simulink model "Q3"  (R2018b)
settings: Solver=FixedStepDiscrete  StartTime=0.0  StopTime=0.1  FixedStep=1e-6  RelTol=1e-3
libraries: powerlib x16
settings Model: Creator=canbe  LastModifiedBy=canbe

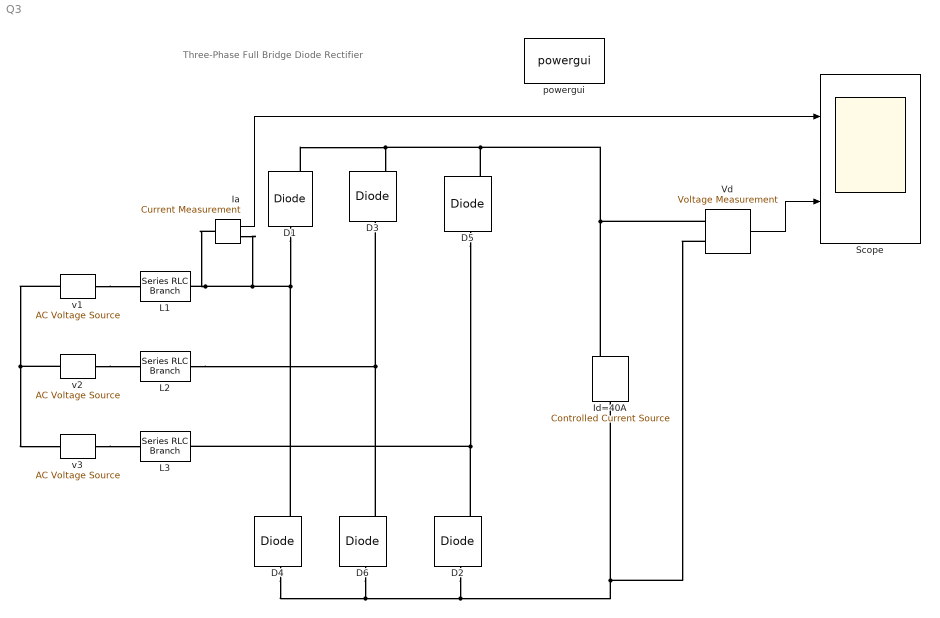
== system Q3 ==
  note: Three-Phase Full Bridge Diode Rectifier
  "D1 " : powerlib/Power Electronics/Diode  Ron=0.001  Lon=0  Vf=0.8  IC=0  UseSnubber=0  Rs=500  Cs=250e-9  Measurements=on
  D2 : powerlib/Power Electronics/Diode  Ron=1e-2  Lon=0  Vf=0.8  IC=0  UseSnubber=off  Rs=1000  Cs=0.1e-6  Measurements=on
      settings: SourceProductName=Simscape Electrical
  "D3 " : powerlib/Power Electronics/Diode  Ron=1e-2  Lon=0  Vf=0.8  IC=0  UseSnubber=off  Rs=1000  Cs=0.1e-6  Measurements=on
      settings: SourceProductName=Simscape Electrical
  "D4 " : powerlib/Power Electronics/Diode  Ron=1e-2  Lon=0  Vf=0.8  IC=0  UseSnubber=off  Rs=1000  Cs=0.1e-6  Measurements=on
      settings: SourceProductName=Simscape Electrical
  "D5 " : powerlib/Power Electronics/Diode  Ron=1e-2  Lon=0  Vf=0.8  IC=0  UseSnubber=off  Rs=1000  Cs=0.1e-6  Measurements=on
      settings: SourceProductName=Simscape Electrical
  D6 : powerlib/Power Electronics/Diode  Ron=1e-2  Lon=0  Vf=0.8  IC=0  UseSnubber=off  Rs=1000  Cs=0.1e-6  Measurements=on
      settings: SourceProductName=Simscape Electrical
  "Ia " : powerlib/Measurements/Current Measurement  PhasorSimulation=off  OutputType=Magnitude  PSBequivalent=0
  "Id=40A " : powerlib/Electrical Sources/Controlled Current Source  Initialize=on  Source_Type=DC  Amplitude=40  Phase=0  Frequency=0  Measurements=None
  L1 : powerlib/Elements/Series RLC Branch  LConnTagsString=__new0  RConnTagsString=__new0  BranchType=L  Resistance=[]  Inductance=1e-3  SetiL0=off  InitialCurrent=0  Capacitance=[]  Setx0=off  InitialVoltage=0  Measurements=None
      settings: SourceProductName=Simscape Electrical
  L2 : powerlib/Elements/Series RLC Branch  LConnTagsString=__new0  RConnTagsString=__new0  BranchType=L  Resistance=[]  Inductance=1e-3  SetiL0=off  InitialCurrent=0  Capacitance=[]  Setx0=off  InitialVoltage=0  Measurements=None
      settings: SourceProductName=Simscape Electrical
  L3 : powerlib/Elements/Series RLC Branch  LConnTagsString=__new0  RConnTagsString=__new0  BranchType=L  Resistance=[]  Inductance=1e-3  SetiL0=off  InitialCurrent=0  Capacitance=[]  Setx0=off  InitialVoltage=0  Measurements=None
      settings: SourceProductName=Simscape Electrical
  Scope : Scope  NumInputPorts=2
  "Vd " : powerlib/Measurements/Voltage Measurement  PhasorSimulation=off  OutputType=Complex  PSBequivalent=0
  powergui : powerlib/powergui  Priority=2  SimulationMode=Discrete  SampleTime=1e-6  frequency=60  Iterations=50  frequencyindice=50  Pbase=100e6  ErrMax=1e-4  UnitsV=kV  UnitsW=MW  buscounter=0  FunctionMessages=off  echomessages=off  EnableUseOfTLC=off  CurrentSourceSwitches=off  DisableSnubberDevices=off  DisableRonSwitches=off  DisableVfSwitches=off  DisplayEquations=off  SolverType=Tustin/Backward Euler (TBE)  Interpol=off  ExternalGateDelay=off  methode=off  Ts=100  x0status=blocks  SPID=off  SwTol=0  HookPort=off  RestoreLinks=warning  ResistiveCurrentMeasurement=off  Frange=[0:2:500]  Ylog=off  Xlog=on  ShowGrid=off  save=off  variable=ZData  structure=0  ZoomFFT=on  StartTime=0.0  cycles=1  DisplayStyle=1  fundamental=60  FreqAxis=off  MaxFrequency=1000  frequencyindicesteady=1  RmsSteady=1  display=off
  v1 : powerlib/Electrical Sources/AC Voltage Source  Description=source block  Amplitude=230*sqrt(2)  Phase=0  Frequency=50  SampleTime=1e-6  Measurements=None  BusType=swing  Pref=10e3  Qref=0  Qmin=-inf  Qmax=+inf
      settings: AttributesFormatString=\n  SourceProductName=Simscape Electrical
  v2 : powerlib/Electrical Sources/AC Voltage Source  Description=source block  Amplitude=230*sqrt(2)  Phase=-120  Frequency=50  SampleTime=1e-6  Measurements=None  BusType=swing  Pref=10e3  Qref=0  Qmin=-inf  Qmax=+inf
      settings: AttributesFormatString=\n  SourceProductName=Simscape Electrical
  v3 : powerlib/Electrical Sources/AC Voltage Source  Description=source block  Amplitude=230*sqrt(2)  Phase=120  Frequency=50  SampleTime=1e-6  Measurements=None  BusType=swing  Pref=10e3  Qref=0  Qmin=-inf  Qmax=+inf
      settings: AttributesFormatString=\n  SourceProductName=Simscape Electrical
  wires:
  "Ia "/1 -> Scope/1
  "Vd "/1 -> Scope/2
  connections:
  L2/RConn1 -- "D3 "/LConn1 -- D6/RConn1
  v1/RConn1 -- L1/LConn1
  v1/LConn1 -- v2/LConn1 -- v3/LConn1
  v2/RConn1 -- L2/LConn1
  v3/RConn1 -- L3/LConn1
  "D1 "/LConn1 -- "D4 "/RConn1 -- "Ia "/RConn1 -- "Ia "/LConn1 -- L1/RConn1
  "D5 "/LConn1 -- D2/RConn1 -- L3/RConn1
  "D4 "/LConn1 -- D6/LConn1 -- "Vd "/LConn2 -- "Id=40A "/RConn1 -- D2/LConn1
  "Id=40A "/LConn1 -- "D5 "/RConn1 -- "D1 "/RConn1 -- "D3 "/RConn1 -- "Vd "/LConn1
